simulink model "diff_eq_system"  (R2019a)
settings: Solver=ode3  StartTime=0.0  StopTime=1000.0  FixedStep=0.001  RelTol=1e-3
model workspace (MAT data in the model file):
  Kb = 0.01
  Kt = 0.001
  La = 0.5
  Ra = 1
libraries: simulink x2
settings Model: OrderedModelArguments=off  Creator=root  LastModifiedBy=dkushn

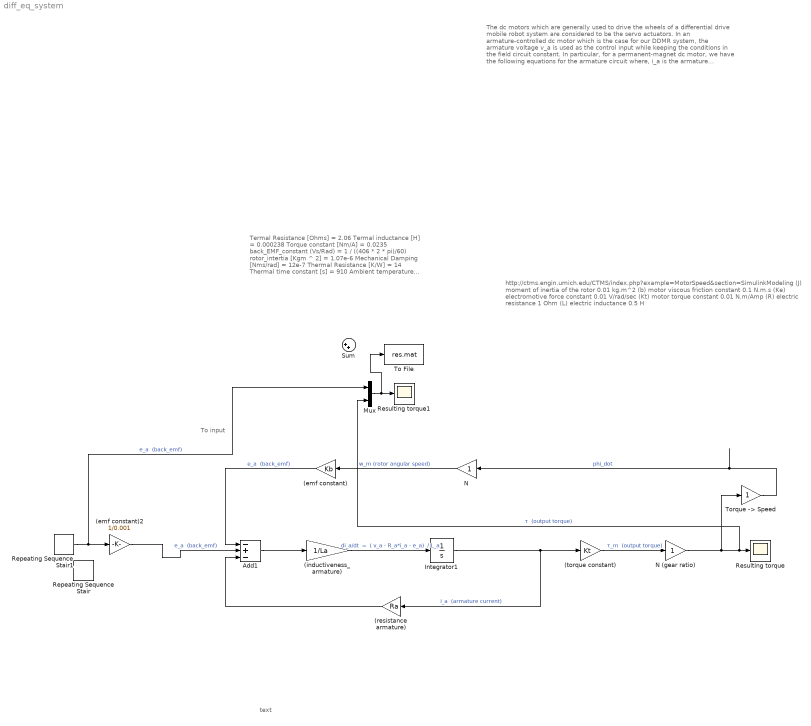
== system diff_eq_system ==
  note: text
  note: To input
  note: http://ctms.engin.umich.edu/CTMS/index.php?example=MotorSpeed&section=SimulinkModeling
      |
      | (J) moment of inertia of the rotor 0.01 kg.m^2
      | (b) motor viscous friction constant 0.1 N.m.s
      | (Ke) electromotive force constant 0.01 V/rad/sec
      | (Kt) motor torque constant 0.01 N.m/Amp
      | (R) electric resistance 1 Ohm
      | (L) electric inductance 0.5 H
  note: Termal Resistance [Ohms] = 2.06
      | Termal inductance [H] = 0.000238
      | Torque constant [Nm/A] = 0.0235
      | back_EMF_constant (Vs/Rad) = 1 / ((406 * 2 * pi)/60)
      | rotor_intertia [Kgm ^ 2] = 1.07e-6
      | Mechanical Damping [Nms/rad] = 12e-7
      | Thermal Resistance [K/W] = 14
      | Thermal time constant [s] = 910
      | Ambient temperature [C] = 22
  note: The dc motors which are generally used to drive the wheels of a differential drive mobile robot system are considered to be the servo actuators. In an armature-controlled dc motor which is the case for our DDMR system, the armature voltage v_a is used as the control input while keeping the conditions in the field circuit constant. In particular, for a permanent-magnet dc motor, we have the following equations for the armature circuit
      |
      | where, i_a is the armature current,(Ra ,La ) is the resistance and inductance of the armature winding respectively, e_a is the back emf, w_m is the rotor angular speed , τ_m is the motor torque, (Kt ,Kb ) are the torque constant and back emf constant respectively, N is the gear ratio, and is τ the output torque applied to the wheel.
      |
      | KD: Rewrite first as:
      | di_a/dt = ( v_a - R_a*i_a - e_a) / L_a
  " (inductiveness_armature)" : Gain  Gain=1/La
  (emf constant) : Gain  Gain=Kb
  (emf constant)2 : Gain  Gain=1/0.001
  (resistance armature) : Gain  Gain=Ra
  (torque constant) : Gain  Gain=Kt
  Add1 : Sum  Inputs=-+-
  Integrator1 : Integrator
  Mux : Mux  Inputs=2
  N : Gain
  N (gear ratio) : Gain
  Repeating Sequence Stair : simulink/Sources/Repeating Sequence Stair  OutValues=[5 10 12 15 8].'  tsamp=10  OutMin=[]  OutMax=[]  OutDataTypeStr=double  OutputDataTypeScalingMode=double  OutDataType=fixdt(0,8)  ConRadixGroup=Best Precision: Vector-wise  OutScaling=2^-12
  Repeating Sequence Stair1 : simulink/Sources/Repeating Sequence Stair  OutValues=[5 10 12 15 8].'  tsamp=7  OutMin=[]  OutMax=[]  OutDataTypeStr=double  OutputDataTypeScalingMode=double  OutDataType=fixdt(0,8)  ConRadixGroup=Best Precision: Vector-wise  OutScaling=2^-12
  Resulting torque : Scope
  Resulting torque1 : Scope
  Sum : Sum  Inputs=|++
  To File : ToFile  Filename=res.mat
  "Torque -> Speed " : Gain
  wires:
  N (gear ratio)/1 -> "Torque -> Speed "/1, Mux/2, Resulting torque/1  "τ  (output torque)"
  (torque constant)/1 -> N (gear ratio)/1  "τ_m  (output torque)"
  (emf constant)/1 -> Add1/1  "e_a  (back_emf)"
  N/1 -> (emf constant)/1  "w_m (rotor angular speed)"
  "Torque -> Speed "/1 -> N/1  "phi_dot"
  Add1/1 -> " (inductiveness_armature)"/1
  Integrator1/1 -> (resistance armature)/1, (torque constant)/1  "i_a  (armature current)"
  (resistance armature)/1 -> Add1/3
  " (inductiveness_armature)"/1 -> Integrator1/1  "di_a/dt  =  ( v_a - R_a*i_a - e_a)  / L_a"
  Mux/1 -> To File/1, Resulting torque1/1
  Repeating Sequence Stair1/1 -> Mux/1, (emf constant)2/1  "e_a  (back_emf)"
  (emf constant)2/1 -> Add1/2  "e_a  (back_emf)"
